simulink model "CanceladorEco"  (R2015a)
settings: Solver=ode45  StartTime=0.0  StopTime=1  RelTol=1e-3
undefined symbols (not defined in the file): Ts
settings Model: Creator=Afonso  LastModifiedBy=Afonso

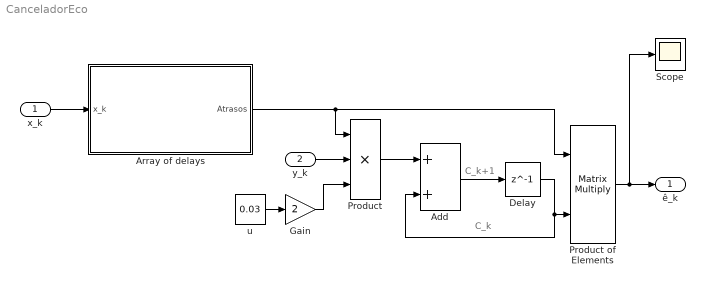
== system CanceladorEco ==
  note: C_k
  note: C_k+1
  x_k : Inport
  y_k : Inport  Port=2
  Add : Sum
  Array of delays : Subsystem
  Delay : Delay  DelayLength=1
  Gain : Gain  Gain=2
  Product : Product  Inputs=3
  Product of Elements : Product  Inputs=**  Multiplication=Matrix(*)
  Scope : Scope
  u : Constant  Value=0.03
  ê_k : Outport
  wires:
  x_k/1 -> Array of delays/1(x_k)
  Array of delays/1(Atrasos) -> Product of Elements/1, Product/1
  y_k/1 -> Product/2
  u/1 -> Gain/1
  Gain/1 -> Product/3
  Product/1 -> Add/1
  Add/1 -> Delay/1
  Delay/1 -> Product of Elements/2, Add/2
  Product of Elements/1 -> ê_k/1, Scope/1

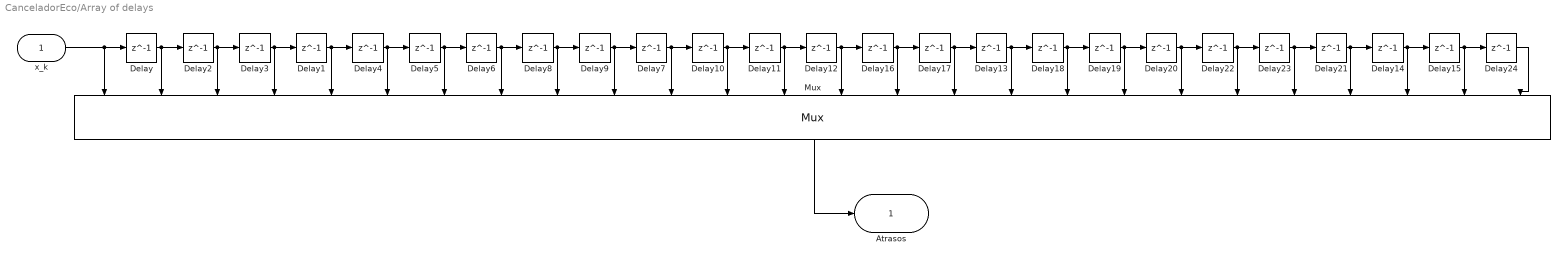
== system CanceladorEco/Array of delays ==
  x_k : Inport
  Delay : Delay  DelayLength=1  SampleTime=Ts
  Delay{1,6..7,12..13,20..21} (7 alike) : Delay  DelayLength=1  SampleTime=0.02
  Delay{2..5,8..11,14..19,22..24} (17 alike) : Delay  DelayLength=1
  Mux : Mux  Inputs=26
  Atrasos : Outport
  wires:
  Delay/1 -> Delay2/1, Mux/2
  Delay2/1 -> Mux/3, Delay3/1
  Delay11/1 -> Mux/13, Delay12/1
  Delay24/1 -> Mux/26
  Delay19/1 -> Delay20/1, Mux/19
  x_k/1 -> Delay/1, Mux/1
  Mux/1 -> Atrasos/1
  Delay15/1 -> Delay24/1, Mux/25
  Delay4/1 -> Mux/6, Delay5/1
  Delay1/1 -> Mux/5, Delay4/1
  Delay5/1 -> Mux/7, Delay6/1
  Delay12/1 -> Mux/14, Delay16/1
  Delay18/1 -> Mux/18, Delay19/1
  Delay16/1 -> Mux/15, Delay17/1
  Delay23/1 -> Delay21/1, Mux/22
  Delay17/1 -> Mux/16, Delay13/1
  Delay22/1 -> Delay23/1, Mux/21
  Delay14/1 -> Delay15/1, Mux/24
  Delay20/1 -> Delay22/1, Mux/20
  Delay13/1 -> Mux/17, Delay18/1
  Delay21/1 -> Delay14/1, Mux/23
  Delay8/1 -> Mux/9, Delay9/1
  Delay6/1 -> Mux/8, Delay8/1
  Delay10/1 -> Delay11/1, Mux/12
  Delay9/1 -> Delay7/1, Mux/10
  Delay7/1 -> Mux/11, Delay10/1
  Delay3/1 -> Mux/4, Delay1/1
